simulink model "Joystick"  (Simulink 7.7)
settings: Solver=ode45  StartTime=0.0  StopTime=inf  FixedStep=sample_time  RelTol=1e-3
InitFcn:
  | sample_time=0.01;
libraries: vrlib x7, simulink_extras x5, HDI_Library x2, nid_lib x2, utility x1
settings Model: Creator=ttcl3  LastModifiedBy=CHIEW
settings SolverCC: MaxConsecutiveMinStep=auto
settings DebuggingCC: MultiTaskRateTransMsg=warning

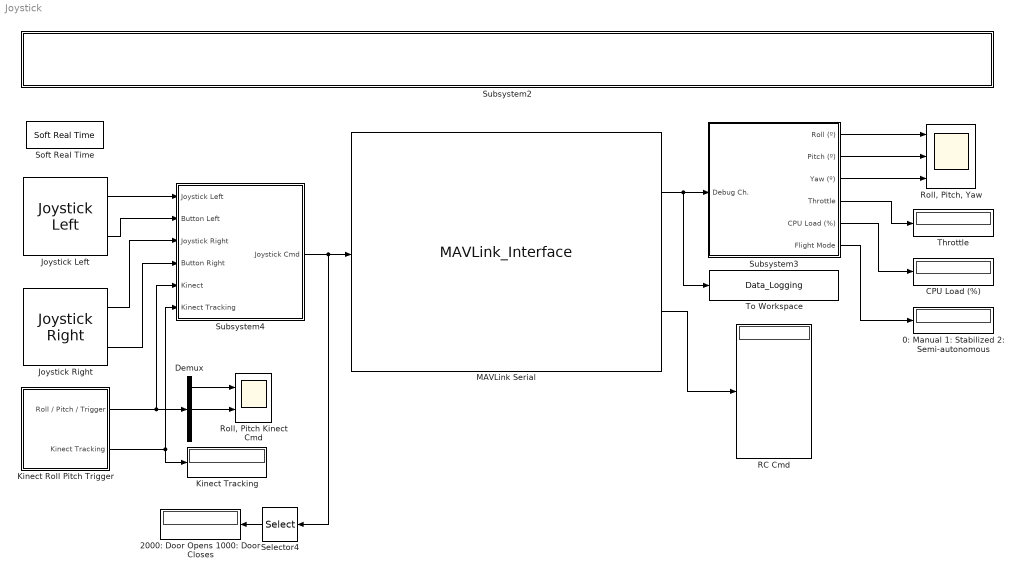
== system Joystick ==
  0: Manual 1: Stabilized 2: Semi-autonomous : Display
  2000: Door Opens 1000: Door Closes : Display
  CPU Load (%) : Display
  Demux : Demux  Outputs=3
  Joystick Left : HDI_Library/Joystick Left  joyid=2  adjustports=on  forcefeed=off
  Joystick Right : HDI_Library/Joystick Right  joyid=1  adjustports=on  forcefeed=off
  Kinect Roll Pitch Trigger : Subsystem
      mask Display: image(imread('kinect.jpg'));port_label('output', 1, 'Roll/Pitch/Trigger'); port_label('output', 2, 'Tracking');
  Kinect Tracking : Display
  MAVLink Serial : S-Function  FunctionName=MAVLink_Interface  Parameters=COM_Port,Baud_Rate,MSG_INPUT,MSG_OUTPUT  EnableBusSupport=off  mask{COM_Port='COM8', Baud_Rate=57600, HEART_BEAT=off, ATTITUDE_OUT=on, RAW_IMU=off, POSITION_OUT=off, VFR_HUD=off, RC_SCALED=on, SERVO_OUT_RAW=off, VICON_XYZ_RPY_Output=off, SET_MODE=off, DATA_STREAM=off, ATTITUDE_COMMAND=off, ATTITUDE_IN=off, GPS_RAW_IN=off, VFR_HUD_IN=off, VICON_XYZ_RPY=on, VICON_VEL=off, POSITION_DESIRED=off}
      mask prompts: COM_Port "COM Port"; Baud_Rate "Baud Rate"; HEART_BEAT "HEART BEAT"; ATTITUDE_OUT "ATTITUDE"; RAW_IMU "RAW IMU"; POSITION_OUT "GLOBAL POSITION"; VFR_HUD "VFR HUD"; RC_SCALED "RC CHANNELS SCALED"; SERVO_OUT_RAW "SERVO OUTPUT RAW"; VICON_XYZ_RPY_Output "VICON Output"; SET_MODE "SET MODE"; DATA_STREAM "REQUEST DATA STREAM"; ATTITUDE_COMMAND "ATTITUDE COMMAND"; ATTITUDE_IN "ATTITUDE (HIL)"; GPS_RAW_IN "GPS RAW (HIL)"; VFR_HUD_IN "AIRSPEED (HIL)"; VICON_XYZ_RPY "VICON POSITION"; VICON_VEL "VICON SPEED"; POSITION_DESIRED "Position Desired"
      mask init:
      | MSG_ID_NUM_INPUT = [uint8(11) uint8(66) uint8(59) uint8(30) uint8(32) uint8(73) uint8(104) uint8(103) uint8(50)];
      | MSG_ID_NAME_INPUT = [SET_MODE DATA_STREAM ATTITUDE_COMMAND ATTITUDE_IN GPS_RAW_IN VFR_HUD_IN VICON_XYZ_RPY VICON_VEL POSITION_DESIRED];
      | 
      | MSG_ID_NUM_OUTPUT = [uint8(0) uint8(30) uint8(27) uint8(73) uint8(74) uint8(34) uint8(37) uint8(104)];
      | MSG_ID_NAME_OUTPUT = [HEART_BEAT ATTITUDE_OUT RAW_IMU VFR_HUD POSITION_OUT RC_SCALED SERVO_OUT_RAW VICON_XYZ_RPY_Output];
      | 
      | idx_input = find(MSG_ID_NAME_INPUT);
      | MSG_INPUT = MSG_ID_NUM_INPUT(idx_input);
      | 
      | idx_output = find(MSG_ID_NAME_OUTPUT);
      | MSG_OUTPUT = MSG_ID_NUM_OUTPUT(idx_output);
      mask TabNameString: Setting,Setting,Output Message,Output Message,Output Message,Output Message,Output Message,Output Message,Output Message,Output Message,Input Message,Input Message,Input Message,Input Message,Input Message,Input Message,Input Message,Input Message,Input Message
      mask Display:
      | % Block image
      | image(imread('10-inch Quad Heat Map.png'));
      | 
      | %Label block
      | fprintf('MAVLink Serial\n%s\n%dbps', COM_Port,  Baud_Rate)
      | 
      | 
      | %Label input ports
      | 
      | in = 1;
      | if (SET_MODE == 1)
      |     port_label('input', in, 'SET MODE');
      |     in = in + 1;
      | end
      | if (DATA_STREAM == 1)
      |     port_label('input', in, 'REQUEST DATA STREAM');
      |     in = in + 1;
      | end
      | if (ATTITUDE_COMMAND == 1)
      |     port_label('input', in, 'ATTITUDE COMMAND');
      |     in = in + 1;
      | end
      | if (ATTITUDE_IN == 1)
      |     port_label('input', in, 'ATTITUDE (HIL)');
      |     in = in + 1;
      | end
      | if (GPS_RAW_IN == 1)
      |     port_label('input', in, 'GPS RAW (HIL)');
      |     in = in + 1;
      | end
      | if (VFR_HUD_IN == 1)
      |     port_label('input', in, 'AIRSPEED (HIL)');
      |     in = in + 1;
      | end
      | if (VICON_XYZ_RPY == 1)
      |     port_label('input', in, 'JOYSTICK CMD');
      |     in = in + 1;
      | end
      | if (VICON_VEL == 1)
      |     port_label('input', in, 'VICON_VEL');
      |     in = in + 1;
      | end
      | 
      | if (POSITION_DESIRED == 1)
      |     port_label('input', in, 'POSITION_DESIRED');
      |     in = in + 1;
      | end
      | 
      | %Label output ports
      | 
      | out = 1;
      | if (HEART_BEAT == 1)
      |     port_label('output', out, 'HEART BEAT');
      |     out = out + 1;
      | end
      | if (ATTITUDE_OUT == 1)
      |     port_label('output', out, 'DEBUG');
      |     out = out + 1;
      | end
      | if (RAW_IMU == 1)
      |     port_label('output', out, 'RAW IMU');
      |     out = out + 1;
      | end
      | if (POSITION_OUT == 1)
      |     port_label('output', out, 'GLOBAL POSITION');
      |     out = out + 1;
      | end
      | if (VFR_HUD == 1)
      |     port_label('output', out, 'VFR HUD');
      |     out = out + 1;
      | end
      | if (RC_SCALED == 1)
      |     port_label('output', out, 'RC CMD');
      |     out = out + 1;
      | end
      | if (SERVO_OUT_RAW == 1)
      |     port_label('output', out, 'SERVO OUTPUT RAW');
      |     out = out + 1;
      | end
      | % weihua, vicon output
      | if (VICON_XYZ_RPY_Output == 1)
      |     port_label('output', out, 'VICON_XYZ_RPY');
      |     out = out + 1;
      | end
  RC Cmd : Display
  "Roll, Pitch Kinect Cmd" : Scope  NumInputPorts=2
      settings: TickLabels=on  TimeRange=24  YMin=-90~-90  YMax=90~90  SampleInput=on
  "Roll, Pitch, Yaw" : Scope  NumInputPorts=3
      settings: TickLabels=on  TimeRange=24  YMin=-90~-90~-90  YMax=90~90~90  SampleInput=on
  Selector4 : Selector  InputPortWidth=7  IndexOptions=Index vector (dialog)  Indices=3  OutputSizes=1
  Soft Real Time : utility/Soft Real Time  x=0.8
  Subsystem2 : Subsystem
      mask Display:
      | %Label block
      | fprintf('NANYANG TECHNOLOGICAL UNIVERSITY')
  Subsystem3 : Subsystem
  Subsystem4 : Subsystem
  Throttle : Display
  To Workspace : ToWorkspace  VariableName=Data_Logging  SampleTime=-1  SaveFormat=Structure With Time
  wires:
  MAVLink Serial/2 -> RC Cmd/1
  Subsystem3/1(Roll (º)) -> "Roll, Pitch, Yaw"/1
  Subsystem3/2(Pitch (º)) -> "Roll, Pitch, Yaw"/2
  Subsystem3/3(Yaw (º)) -> "Roll, Pitch, Yaw"/3
  Subsystem3/4(Throttle) -> Throttle/1
  Subsystem3/5(CPU Load (%)) -> CPU Load (%)/1
  Subsystem3/6(Flight Mode) -> 0: Manual 1: Stabilized 2: Semi-autonomous/1
  MAVLink Serial/1 -> Subsystem3/1(Debug Ch.), To Workspace/1
  Subsystem4/1(Joystick Cmd) -> MAVLink Serial/1, Selector4/1
  Kinect Roll Pitch Trigger/1(Roll / Pitch / Trigger) -> Subsystem4/5(Kinect), Demux/1
  Selector4/1 -> 2000: Door Opens 1000: Door Closes/1
  Kinect Roll Pitch Trigger/2(Kinect Tracking) -> Kinect Tracking/1, Subsystem4/6(Kinect Tracking)
  Demux/1 -> "Roll, Pitch Kinect Cmd"/1
  Demux/2 -> "Roll, Pitch Kinect Cmd"/2
  Joystick Right/1 -> Subsystem4/3(Joystick Right)
  Joystick Right/2 -> Subsystem4/4(Button Right)
  Joystick Left/1 -> Subsystem4/1(Joystick Left)
  Joystick Left/2 -> Subsystem4/2(Button Left)

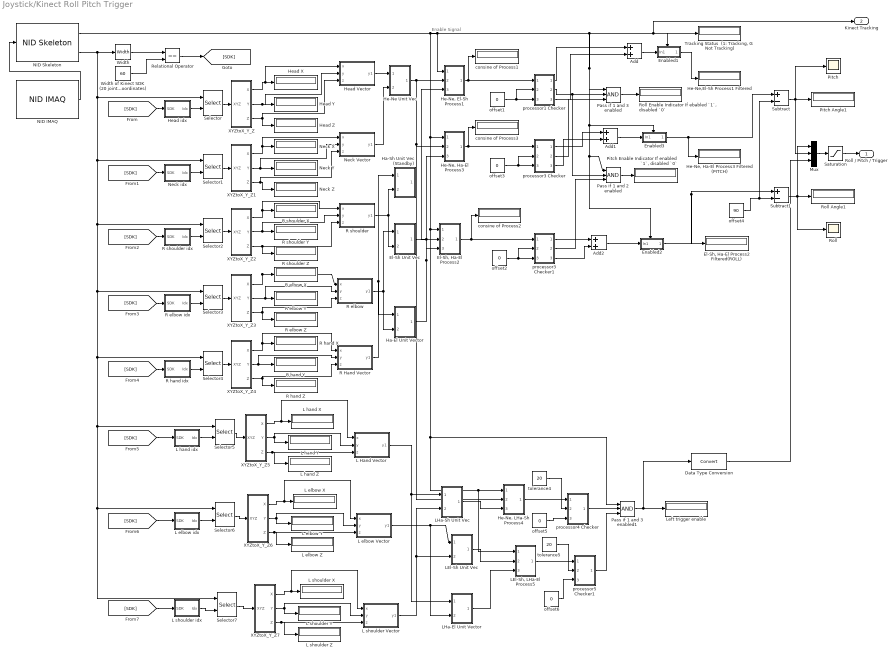
== system Joystick/Kinect Roll Pitch Trigger ==
  note: Enable Signal
  Add : Sum
  Add1 : Sum
  Add2 : Sum
  Data Type Conversion : DataTypeConversion
  El-Sh Unit Vec : Subsystem
  "El-Sh, Ha-El Process2" : Subsystem
  "El-Sh, Ha-El Process2 Filtered(ROLL)" : Display
  Enabled1 : Subsystem  TreatAsAtomicUnit=on
  Enabled2 : Subsystem  TreatAsAtomicUnit=on
  Enabled3 : Subsystem  TreatAsAtomicUnit=on
  Ha-El Unit Vector : Subsystem
  Ha-Sh Unit Vec (Standby) : Subsystem
  He-Ne Unit Vec : Subsystem
  "He-Ne, El-Sh Process1" : Subsystem
  "He-Ne, Ha-El Process3" : Subsystem
  "He-Ne, Ha-El Process3 Filtered (PITCH)" : Display
  "He-Ne, LHa-Sh Process4" : Subsystem
  "He-Ne,El-Sh Process1 Filtered " : Display
  Head Vector : Stateflow chart  TreatAsAtomicUnit=on
  Head X : Display
  Head Y : Display
  Head Z : Display
  Head idx : Subsystem
  L Hand Vector : Stateflow chart  TreatAsAtomicUnit=on
  L elbow Vector : Stateflow chart  TreatAsAtomicUnit=on
  L elbow X : Display
  L elbow Y : Display
  L elbow Z : Display
  L elbow idx : Subsystem
  L hand X : Display
  L hand Y : Display
  L hand Z : Display
  L hand idx : Subsystem
  L shoulder Vector : Stateflow chart  TreatAsAtomicUnit=on
  L shoulder X : Display
  L shoulder Y : Display
  L shoulder Z : Display
  L shoulder idx : Subsystem
  LEl-Sh Unit Vec : Subsystem
  "LEl-Sh, LHa-El Process5" : Subsystem
  LHa-El Unit Vector : Subsystem
  LHa-Sh Unit Vec : Subsystem
  Left trigger enable : Display
  Mux : Mux  Inputs=3
  NID IMAQ : nid_lib/NID IMAQ  imaq_depth=off  imaq_motion=off  imaq_image=off  view_point=off  imaq_skeleton=on  imaq_ir=off  mirror_image=off  imaq_sample_time=1/30  res_fps=VGA (640x480): 30 FPS  needPsiPose=off  angle_input=off  angle=0  angle_read=off  near_mode=off  seated_mode=off  skeleton_smooth=[0.5 0.5 0.5 0.05 0.04]  infer_skeleton=on
  NID Skeleton : nid_lib/NID Skeleton  num_of_skeleton_tracking=1  conv_XYZ_RW=on  viewer=off
  Neck Vector : Stateflow chart  TreatAsAtomicUnit=on
  Neck X : Display
  Neck Y : Display
  Neck Z : Display
  Neck idx : Subsystem
  Pass if 1 and 2 enabled : Logic  Inputs=3  AllPortsSameDT=off  OutDataTypeStr=boolean
  Pass if 1 and 3 enabled : Logic  Inputs=3  AllPortsSameDT=off  OutDataTypeStr=boolean
  Pass if 1 and 3 enabled1 : Logic  Inputs=3  AllPortsSameDT=off  OutDataTypeStr=boolean
  Pitch : Scope
      settings: YMin=-90  YMax=90  SaveName=ScopeData3
  Pitch Angle1 : Display
  "Pitch Enable Indicator If enabled `1`, disabled `0` " : Display
  R Hand Vector : Stateflow chart  TreatAsAtomicUnit=on
  R elbow : Stateflow chart  TreatAsAtomicUnit=on
  R elbow X : Display
  R elbow Y : Display
  R elbow Z : Display
  R elbow idx : Subsystem
  R hand X : Display
  R hand Y : Display
  R hand Z : Display
  R hand idx : Subsystem
  R shoulder : Stateflow chart  TreatAsAtomicUnit=on
  R shoulder X : Display
  R shoulder Y : Display
  R shoulder Z : Display
  R shoulder idx : Subsystem
  Relational Operator : RelationalOperator  Operator===  OutDataTypeStr=boolean
  Roll : Scope
      settings: YMin=-90  YMax=90  SaveName=ScopeData2
  Roll Angle1 : Display
  "Roll Enable Indicator If ebabled `1`, disabled `0`" : Display
  Saturation : Saturate  UpperLimit=30  LowerLimit=-30
  Selector{,1..7} (8 alike) : Selector  NumberOfDimensions=3  InputPortWidth=3  IndexOptions=Select all,Index vector (port),Select all  Indices=[1 3],1,1  OutputSizes=1,1,1
  Subtract : Sum  Inputs=+-
  Subtract1 : Sum  Inputs=+-
  "Tracking Status  (1: Tracking, 0: Not Tracking)" : Display
  Width : Width
  Width of Kinect SDK  (20 joints x 3 coordinates) : Constant  Value=60
  XYZtoX_Y_Z : Subsystem
  XYZtoX_Y_Z1 : Subsystem
  XYZtoX_Y_Z2 : Subsystem
  XYZtoX_Y_Z3 : Subsystem
  XYZtoX_Y_Z4 : Subsystem
  XYZtoX_Y_Z5 : Subsystem
  XYZtoX_Y_Z6 : Subsystem
  XYZtoX_Y_Z7 : Subsystem
  consine of Process1 : Display
  consine of Process2 : Display
  consine of Process3 : Display
  offset{1..3,5..6} (5 alike) : Constant  Value=0
  offset4 : Constant  Value=90
  processor1 Checker : Subsystem
  processor3 Checker : Subsystem
  processor3 Checker1 : Subsystem
  processor4 Checker : Subsystem
  processor5 Checker1 : Subsystem
  tolerance4 : Constant  Value=20
  tolerance5 : Constant  Value=20
  Roll / Pitch / Trigger : Outport
  Kinect Tracking : Outport  Port=2
  wires:
  Saturation/1 -> Roll / Pitch / Trigger/1
  Mux/1 -> Saturation/1
  Pass if 1 and 3 enabled/1 -> "Roll Enable Indicator If ebabled `1`, disabled `0`"/1
  Subtract1/1 -> Roll/1, Mux/1, Roll Angle1/1
  Subtract/1 -> Pitch/1, Mux/2, Pitch Angle1/1
  offset4/1 -> Subtract/2, Subtract1/2
  Add2/1 -> Enabled2/1(In1)
  processor3 Checker1/3(Out3) -> Add2/2
  processor3 Checker1/1(Out1) -> Add2/1
  processor3 Checker/3(Out3) -> Add1/2
  processor3 Checker/1(Out1) -> Add1/1
  Add1/1 -> Enabled3/1(In1)
  processor1 Checker/1(Out1) -> Add/1
  Add/1 -> Enabled1/1(In1)
  processor1 Checker/3(Out3) -> Add/2
  Enabled2/1(Out1) -> Subtract1/1, "El-Sh, Ha-El Process2 Filtered(ROLL)"/1
  Enabled1/1(Out1) -> "He-Ne,El-Sh Process1 Filtered "/1
  Enabled3/1(Out1) -> Subtract/1, "He-Ne, Ha-El Process3 Filtered (PITCH)"/1
  offset2/1 -> processor3 Checker1/2(In2), processor3 Checker1/3(In3)
  offset3/1 -> processor3 Checker/2(In2), processor3 Checker/3(In3)
  offset1/1 -> processor1 Checker/2(In2), processor1 Checker/3(In3)
  processor3 Checker1/2(Out2) -> Pass if 1 and 2 enabled/3
  processor1 Checker/2(Out2) -> Pass if 1 and 2 enabled/2, Pass if 1 and 3 enabled/2
  processor3 Checker/2(Out2) -> Pass if 1 and 3 enabled/3
  Pass if 1 and 2 enabled/1 -> "Pitch Enable Indicator If enabled `1`, disabled `0` "/1
  "El-Sh, Ha-El Process2"/1(Out1) -> processor3 Checker1/1(In1), consine of Process2/1
  "He-Ne, El-Sh Process1"/1(Out1) -> consine of Process1/1, processor1 Checker/1(In1)
  "He-Ne, Ha-El Process3"/1(Out1) -> processor3 Checker/1(In1), consine of Process3/1
  Ha-El Unit Vector/1(Out1) -> "He-Ne, Ha-El Process3"/3(In3), "El-Sh, Ha-El Process2"/3(In3)
  El-Sh Unit Vec/1(Out1) -> "El-Sh, Ha-El Process2"/2(In2), "He-Ne, El-Sh Process1"/3(In3)
  He-Ne Unit Vec/1(Out1) -> "He-Ne, El-Sh Process1"/2(In2), "He-Ne, Ha-El Process3"/2(In2), "He-Ne, LHa-Sh Process4"/2(In2)
  R elbow/1(y1) -> Ha-El Unit Vector/2(In2), El-Sh Unit Vec/1(In1)
  R Hand Vector/1(y1) -> Ha-El Unit Vector/1(In1), Ha-Sh Unit Vec (Standby)/1(In1)
  R shoulder/1(y1) -> El-Sh Unit Vec/2(In2), Ha-Sh Unit Vec (Standby)/2(In2)
  Head Vector/1(y1) -> He-Ne Unit Vec/1(In1)
  Neck Vector/1(y1) -> He-Ne Unit Vec/2(In2)
  Selector/1 -> XYZtoX_Y_Z/1(XYZ)
  Selector4/1 -> XYZtoX_Y_Z4/1(XYZ)
  XYZtoX_Y_Z4/3(Z) -> R Hand Vector/3(z), R hand Z/1
  XYZtoX_Y_Z4/2(Y) -> R Hand Vector/2(y), R hand Y/1
  XYZtoX_Y_Z4/1(X) -> R Hand Vector/1(x), R hand X/1
  Selector3/1 -> XYZtoX_Y_Z3/1(XYZ)
  XYZtoX_Y_Z3/3(Z) -> R elbow/3(z), R elbow Z/1
  XYZtoX_Y_Z3/2(Y) -> R elbow/2(y), R elbow Y/1
  XYZtoX_Y_Z3/1(X) -> R elbow/1(x), R elbow X/1
  Selector2/1 -> XYZtoX_Y_Z2/1(XYZ)
  XYZtoX_Y_Z2/3(Z) -> R shoulder/3(z), R shoulder Z/1
  XYZtoX_Y_Z2/2(Y) -> R shoulder/2(y), R shoulder Y/1
  XYZtoX_Y_Z2/1(X) -> R shoulder/1(x), R shoulder X/1
  XYZtoX_Y_Z1/3(Z) -> Neck Vector/3(z), Neck Z/1
  XYZtoX_Y_Z1/2(Y) -> Neck Vector/2(y), Neck Y/1
  XYZtoX_Y_Z1/1(X) -> Neck Vector/1(x), Neck X/1
  XYZtoX_Y_Z/3(Z) -> Head Vector/3(z), Head Z/1
  XYZtoX_Y_Z/2(Y) -> Head Vector/2(y), Head Y/1
  [SDK] -> R hand idx/1(SDK)
  R hand idx/1(Idx) -> Selector4/2
  [SDK] -> R elbow idx/1(SDK)
  R elbow idx/1(Idx) -> Selector3/2
  [SDK] -> R shoulder idx/1(SDK)
  R shoulder idx/1(Idx) -> Selector2/2
  Selector1/1 -> XYZtoX_Y_Z1/1(XYZ)
  [SDK] -> Neck idx/1(SDK)
  Neck idx/1(Idx) -> Selector1/2
  XYZtoX_Y_Z/1(X) -> Head Vector/1(x), Head X/1
  NID Skeleton/1 -> "He-Ne, El-Sh Process1"/1(In1), Pass if 1 and 3 enabled/1, Kinect Tracking/1, "Tracking Status  (1: Tracking, 0: Not Tracking)"/1, Enabled1/Enable, Enabled3/Enable, Enabled2/Enable, Pass if 1 and 2 enabled/1, "He-Ne, Ha-El Process3"/1(In1), "El-Sh, Ha-El Process2"/1(In1), "He-Ne, LHa-Sh Process4"/1(In1), "LEl-Sh, LHa-El Process5"/1(In1), Pass if 1 and 3 enabled1/1
  [SDK] -> Head idx/1(SDK)
  Head idx/1(Idx) -> Selector/2
  Relational Operator/1 -> [SDK]
  NID Skeleton/2 -> Selector3/1, Selector4/1, Selector5/1, Selector6/1, Selector7/1, Selector2/1, Selector1/1, Selector/1, Width/1
  Width of Kinect SDK  (20 joints x 3 coordinates)/1 -> Relational Operator/2
  Width/1 -> Relational Operator/1
  NID IMAQ/1 -> NID Skeleton/1
  [SDK] -> L hand idx/1(SDK)
  [SDK] -> L elbow idx/1(SDK)
  [SDK] -> L shoulder idx/1(SDK)
  L hand idx/1(Idx) -> Selector5/2
  L elbow idx/1(Idx) -> Selector6/2
  L shoulder idx/1(Idx) -> Selector7/2
  Selector5/1 -> XYZtoX_Y_Z5/1(XYZ)
  XYZtoX_Y_Z5/1(X) -> L hand X/1, L Hand Vector/1(x)
  XYZtoX_Y_Z5/2(Y) -> L hand Y/1, L Hand Vector/2(y)
  XYZtoX_Y_Z5/3(Z) -> L hand Z/1, L Hand Vector/3(z)
  XYZtoX_Y_Z6/1(X) -> L elbow X/1, L elbow Vector/1(x)
  XYZtoX_Y_Z6/2(Y) -> L elbow Y/1, L elbow Vector/2(y)
  XYZtoX_Y_Z6/3(Z) -> L elbow Z/1, L elbow Vector/3(z)
  XYZtoX_Y_Z7/1(X) -> L shoulder X/1, L shoulder Vector/1(x)
  XYZtoX_Y_Z7/2(Y) -> L shoulder Y/1, L shoulder Vector/2(y)
  XYZtoX_Y_Z7/3(Z) -> L shoulder Z/1, L shoulder Vector/3(z)
  Selector6/1 -> XYZtoX_Y_Z6/1(XYZ)
  L Hand Vector/1(y1) -> LHa-Sh Unit Vec/1(In1), LHa-El Unit Vector/1(In1)
  L shoulder Vector/1(y1) -> LHa-Sh Unit Vec/2(In2), LEl-Sh Unit Vec/2(In2)
  LHa-Sh Unit Vec/1(Out1) -> "He-Ne, LHa-Sh Process4"/3(In3)
  "He-Ne, LHa-Sh Process4"/1(Out1) -> processor4 Checker/1(In1)
  tolerance4/1 -> processor4 Checker/2(In2)
  offset5/1 -> processor4 Checker/3(In3)
  Selector7/1 -> XYZtoX_Y_Z7/1(XYZ)
  processor4 Checker/1(Out2) -> Pass if 1 and 3 enabled1/2
  L elbow Vector/1(y1) -> LEl-Sh Unit Vec/1(In1), LHa-El Unit Vector/2(In2)
  LEl-Sh Unit Vec/1(Out1) -> "LEl-Sh, LHa-El Process5"/2(In2)
  LHa-El Unit Vector/1(Out1) -> "LEl-Sh, LHa-El Process5"/3(In3)
  "LEl-Sh, LHa-El Process5"/1(Out1) -> processor5 Checker1/1(In1)
  tolerance5/1 -> processor5 Checker1/2(In2)
  offset6/1 -> processor5 Checker1/3(In3)
  processor5 Checker1/1(Out2) -> Pass if 1 and 3 enabled1/3
  Pass if 1 and 3 enabled1/1 -> Left trigger enable/1, Data Type Conversion/1
  Data Type Conversion/1 -> Mux/3

== system Joystick/Subsystem2 ==

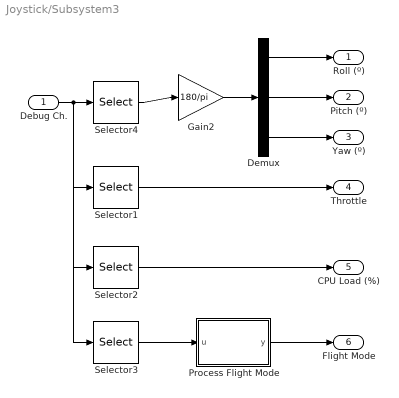
== system Joystick/Subsystem3 ==
  Debug Ch. : Inport
  Demux : Demux  Outputs=3
  Gain2 : Gain  Gain=180/pi
  Process Flight Mode : Stateflow chart  TreatAsAtomicUnit=on
  Selector1 : Selector  InputPortWidth=6  IndexOptions=Index vector (dialog)  Indices=4  OutputSizes=1
  Selector2 : Selector  InputPortWidth=6  IndexOptions=Index vector (dialog)  Indices=5  OutputSizes=1
  Selector3 : Selector  InputPortWidth=6  IndexOptions=Index vector (dialog)  Indices=6  OutputSizes=1
  Selector4 : Selector  InputPortWidth=6  IndexOptions=Index vector (dialog)  Indices=[1 2 3]  OutputSizes=1
  Roll (º) : Outport
  Pitch (º) : Outport  Port=2
  Yaw (º) : Outport  Port=3
  Throttle : Outport  Port=4
  CPU Load (%) : Outport  Port=5
  Flight Mode : Outport  Port=6
  wires:
  Selector4/1 -> Gain2/1
  Gain2/1 -> Demux/1
  Demux/1 -> Roll (º)/1
  Demux/2 -> Pitch (º)/1
  Debug Ch./1 -> Selector4/1, Selector1/1, Selector2/1, Selector3/1
  Demux/3 -> Yaw (º)/1
  Selector1/1 -> Throttle/1
  Selector2/1 -> CPU Load (%)/1
  Selector3/1 -> Process Flight Mode/1(u)
  Process Flight Mode/1(y) -> Flight Mode/1

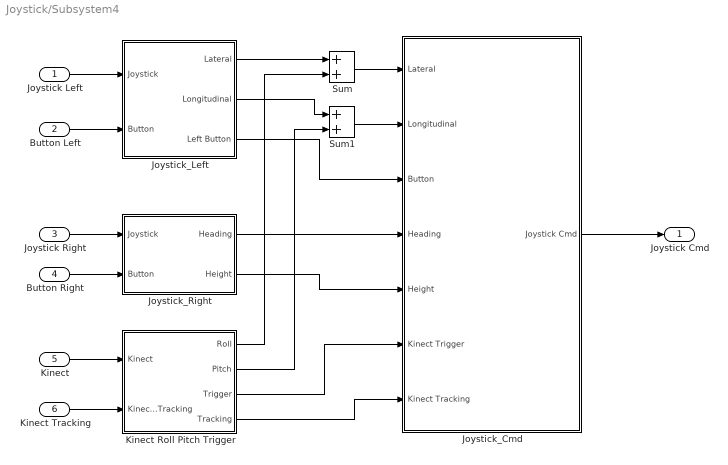
== system Joystick/Subsystem4 ==
  Joystick Left : Inport
  Button Left : Inport  Port=2
  Joystick Right : Inport  Port=3
  Button Right : Inport  Port=4
  Kinect : Inport  Port=5
  Kinect Tracking : Inport  Port=6
  Joystick_Cmd : Subsystem
  Joystick_Left : Subsystem
  Joystick_Right : Subsystem
  Kinect Roll Pitch Trigger : Subsystem
  Sum : Sum
  Sum1 : Sum
  Joystick Cmd : Outport
  wires:
  Joystick Left/1 -> Joystick_Left/1(Joystick)
  Joystick Right/1 -> Joystick_Right/1(Joystick)
  Button Right/1 -> Joystick_Right/2(Button)
  Button Left/1 -> Joystick_Left/2(Button)
  Joystick_Right/1(Heading) -> Joystick_Cmd/4(Heading)
  Joystick_Right/2(Height) -> Joystick_Cmd/5(Height)
  Kinect/1 -> Kinect Roll Pitch Trigger/1(Kinect)
  Joystick_Left/3(Left Button) -> Joystick_Cmd/3(Button)
  Joystick_Cmd/1(Joystick Cmd) -> Joystick Cmd/1
  Joystick_Left/1(Lateral) -> Sum/1
  Sum/1 -> Joystick_Cmd/1(Lateral)
  Sum1/1 -> Joystick_Cmd/2(Longitudinal)
  Joystick_Left/2(Longitudinal) -> Sum1/1
  Kinect Roll Pitch Trigger/3(Trigger) -> Joystick_Cmd/6(Kinect Trigger)
  Kinect Tracking/1 -> Kinect Roll Pitch Trigger/2(Kinect Tracking)
  Kinect Roll Pitch Trigger/4(Tracking) -> Joystick_Cmd/7(Kinect Tracking)
  Kinect Roll Pitch Trigger/1(Roll) -> Sum/2
  Kinect Roll Pitch Trigger/2(Pitch) -> Sum1/2

== system Joystick/Kinect Roll Pitch Trigger/El-Sh Unit Vec ==
  In1 : Inport
  In2 : Inport  Port=2
  Shoudler Elbow : vrlib/Utilities/Normalize Vector  SystemSampleTime=-1  maxzero=0
  Subtract3 : Sum  Inputs=+-
  Out1 : Outport
  wires:
  Shoudler Elbow/1 -> Out1/1
  In2/1 -> Subtract3/2
  In1/1 -> Subtract3/1
  Subtract3/1 -> Shoudler Elbow/1

== system Joystick/Kinect Roll Pitch Trigger/El-Sh, Ha-El Process2 ==
  In1 : Inport
  In2 : Inport  Port=2
  In3 : Inport  Port=3
  Enabled Subsystem2 : Subsystem  TreatAsAtomicUnit=on
  "consine El-Sh, Ha-El" : DotProduct  InputSameDT=on  OutDataTypeStr=Inherit: Inherit via internal rule
  Out1 : Outport
  wires:
  Enabled Subsystem2/1(Out1) -> Out1/1
  In3/1 -> "consine El-Sh, Ha-El"/2
  In2/1 -> "consine El-Sh, Ha-El"/1
  In1/1 -> Enabled Subsystem2/Enable
  "consine El-Sh, Ha-El"/1 -> Enabled Subsystem2/1(In1)

== system Joystick/Kinect Roll Pitch Trigger/Enabled1 ==
  In1 : Inport
  Enable : EnablePort
  Out1 : Outport
  wires:
  In1/1 -> Out1/1

== system Joystick/Kinect Roll Pitch Trigger/Enabled2 ==
  In1 : Inport
  Enable : EnablePort
  Out1 : Outport
  wires:
  In1/1 -> Out1/1

== system Joystick/Kinect Roll Pitch Trigger/Enabled3 ==
  In1 : Inport
  Enable : EnablePort
  Out1 : Outport
  wires:
  In1/1 -> Out1/1

== system Joystick/Kinect Roll Pitch Trigger/Ha-El Unit Vector ==
  In1 : Inport
  In2 : Inport  Port=2
  Elbow Hand : vrlib/Utilities/Normalize Vector  SystemSampleTime=-1  maxzero=0
  Subtract2 : Sum  Inputs=+-
  Out1 : Outport
  wires:
  Elbow Hand/1 -> Out1/1
  In2/1 -> Subtract2/2
  In1/1 -> Subtract2/1
  Subtract2/1 -> Elbow Hand/1

== system Joystick/Kinect Roll Pitch Trigger/Ha-Sh Unit Vec (Standby) ==
  In1 : Inport
  In2 : Inport  Port=2
  Subtract1 : Sum  Inputs=+-
  Unit Vector1 : vrlib/Utilities/Normalize Vector  SystemSampleTime=-1  maxzero=0
  Out1 : Outport
  wires:
  Unit Vector1/1 -> Out1/1
  In2/1 -> Subtract1/2
  In1/1 -> Subtract1/1
  Subtract1/1 -> Unit Vector1/1

== system Joystick/Kinect Roll Pitch Trigger/He-Ne Unit Vec ==
  In1 : Inport
  In2 : Inport  Port=2
  Subtract : Sum  Inputs=+-
  Unit Vector : vrlib/Utilities/Normalize Vector  SystemSampleTime=-1  maxzero=0
  Out1 : Outport
  wires:
  In2/1 -> Subtract/2
  Unit Vector/1 -> Out1/1
  In1/1 -> Subtract/1
  Subtract/1 -> Unit Vector/1

== system Joystick/Kinect Roll Pitch Trigger/He-Ne, El-Sh Process1 ==
  In1 : Inport
  In2 : Inport  Port=2
  In3 : Inport  Port=3
  Enabled Subsystem1 : Subsystem  TreatAsAtomicUnit=on
  consine He-Ne El-Sh : DotProduct  InputSameDT=on  OutDataTypeStr=Inherit: Inherit via internal rule
  Out1 : Outport
  wires:
  Enabled Subsystem1/1(Out1) -> Out1/1
  In3/1 -> consine He-Ne El-Sh/2
  In2/1 -> consine He-Ne El-Sh/1
  In1/1 -> Enabled Subsystem1/Enable
  consine He-Ne El-Sh/1 -> Enabled Subsystem1/1(In1)

== system Joystick/Kinect Roll Pitch Trigger/He-Ne, Ha-El Process3 ==
  In1 : Inport
  In2 : Inport  Port=2
  In3 : Inport  Port=3
  Enabled Subsystem3 : Subsystem  TreatAsAtomicUnit=on
  "consine He-Ne, Ha-El" : DotProduct  InputSameDT=on  OutDataTypeStr=Inherit: Inherit via internal rule
  Out1 : Outport
  wires:
  Enabled Subsystem3/1(Out1) -> Out1/1
  In3/1 -> "consine He-Ne, Ha-El"/2
  In2/1 -> "consine He-Ne, Ha-El"/1
  In1/1 -> Enabled Subsystem3/Enable
  "consine He-Ne, Ha-El"/1 -> Enabled Subsystem3/1(In1)

== system Joystick/Kinect Roll Pitch Trigger/He-Ne, LHa-Sh Process4 ==
  In1 : Inport
  In2 : Inport  Port=2
  In3 : Inport  Port=3
  Enabled Subsystem1 : Subsystem  TreatAsAtomicUnit=on
  consine He-Ne El-Sh : DotProduct  InputSameDT=on  OutDataTypeStr=Inherit: Inherit via internal rule
  Out1 : Outport
  wires:
  consine He-Ne El-Sh/1 -> Enabled Subsystem1/1(In1)
  In1/1 -> Enabled Subsystem1/Enable
  In2/1 -> consine He-Ne El-Sh/1
  In3/1 -> consine He-Ne El-Sh/2
  Enabled Subsystem1/1(Out1) -> Out1/1

== system Joystick/Kinect Roll Pitch Trigger/Head idx ==
  SDK : Inport
  Kinect SDK : Constant  Value=4
  OpenNI : Constant
  Switch : Switch  Criteria=u2 ~= 0
  Idx : Outport
  wires:
  Switch/1 -> Idx/1
  SDK/1 -> Switch/2
  OpenNI/1 -> Switch/3
  Kinect SDK/1 -> Switch/1

== system Joystick/Kinect Roll Pitch Trigger/L elbow idx ==
  SDK : Inport
  Kinect SDK : Constant  Value=6
  OpenNI : Constant  Value=8
  Switch : Switch  Criteria=u2 ~= 0
  Idx : Outport
  wires:
  Kinect SDK/1 -> Switch/1
  OpenNI/1 -> Switch/3
  SDK/1 -> Switch/2
  Switch/1 -> Idx/1

== system Joystick/Kinect Roll Pitch Trigger/L hand idx ==
  SDK : Inport
  Kinect SDK : Constant  Value=8
  OpenNI : Constant  Value=9
  Switch : Switch  Criteria=u2 ~= 0
  Idx : Outport
  wires:
  Kinect SDK/1 -> Switch/1
  OpenNI/1 -> Switch/3
  SDK/1 -> Switch/2
  Switch/1 -> Idx/1

== system Joystick/Kinect Roll Pitch Trigger/L shoulder idx ==
  SDK : Inport
  Kinect SDK : Constant  Value=5
  OpenNI : Constant  Value=7
  Switch : Switch  Criteria=u2 ~= 0
  Idx : Outport
  wires:
  Kinect SDK/1 -> Switch/1
  OpenNI/1 -> Switch/3
  SDK/1 -> Switch/2
  Switch/1 -> Idx/1

== system Joystick/Kinect Roll Pitch Trigger/LEl-Sh Unit Vec ==
  In1 : Inport
  In2 : Inport  Port=2
  Shoudler Elbow : vrlib/Utilities/Normalize Vector  SystemSampleTime=-1  maxzero=0
  Subtract3 : Sum  Inputs=+-
  Out1 : Outport
  wires:
  Subtract3/1 -> Shoudler Elbow/1
  In1/1 -> Subtract3/1
  In2/1 -> Subtract3/2
  Shoudler Elbow/1 -> Out1/1

== system Joystick/Kinect Roll Pitch Trigger/LEl-Sh, LHa-El Process5 ==
  In1 : Inport
  In2 : Inport  Port=2
  In3 : Inport  Port=3
  Enabled Subsystem2 : Subsystem  TreatAsAtomicUnit=on
  "consine El-Sh, Ha-El" : DotProduct  InputSameDT=on  OutDataTypeStr=Inherit: Inherit via internal rule
  Out1 : Outport
  wires:
  "consine El-Sh, Ha-El"/1 -> Enabled Subsystem2/1(In1)
  In1/1 -> Enabled Subsystem2/Enable
  In2/1 -> "consine El-Sh, Ha-El"/1
  In3/1 -> "consine El-Sh, Ha-El"/2
  Enabled Subsystem2/1(Out1) -> Out1/1

== system Joystick/Kinect Roll Pitch Trigger/LHa-El Unit Vector ==
  In1 : Inport
  In2 : Inport  Port=2
  Elbow Hand : vrlib/Utilities/Normalize Vector  SystemSampleTime=-1  maxzero=0
  Subtract2 : Sum  Inputs=+-
  Out1 : Outport
  wires:
  Subtract2/1 -> Elbow Hand/1
  In1/1 -> Subtract2/1
  In2/1 -> Subtract2/2
  Elbow Hand/1 -> Out1/1

== system Joystick/Kinect Roll Pitch Trigger/LHa-Sh Unit Vec ==
  In1 : Inport
  In2 : Inport  Port=2
  Subtract1 : Sum  Inputs=+-
  Unit Vector1 : vrlib/Utilities/Normalize Vector  SystemSampleTime=-1  maxzero=0
  Out1 : Outport
  wires:
  Subtract1/1 -> Unit Vector1/1
  In1/1 -> Subtract1/1
  In2/1 -> Subtract1/2
  Unit Vector1/1 -> Out1/1

== system Joystick/Kinect Roll Pitch Trigger/Neck idx ==
  SDK : Inport
  Kinect SDK : Constant  Value=3
  OpenNI : Constant  Value=2
  Switch : Switch  Criteria=u2 ~= 0
  Idx : Outport
  wires:
  Kinect SDK/1 -> Switch/1
  OpenNI/1 -> Switch/3
  SDK/1 -> Switch/2
  Switch/1 -> Idx/1

== system Joystick/Kinect Roll Pitch Trigger/R elbow idx ==
  SDK : Inport
  Kinect SDK : Constant  Value=10
  OpenNI : Constant  Value=5
  Switch : Switch  Criteria=u2 ~= 0
  Idx : Outport
  wires:
  Switch/1 -> Idx/1
  SDK/1 -> Switch/2
  OpenNI/1 -> Switch/3
  Kinect SDK/1 -> Switch/1

== system Joystick/Kinect Roll Pitch Trigger/R hand idx ==
  SDK : Inport
  Kinect SDK : Constant  Value=12
  OpenNI : Constant  Value=6
  Switch : Switch  Criteria=u2 ~= 0
  Idx : Outport
  wires:
  Switch/1 -> Idx/1
  SDK/1 -> Switch/2
  OpenNI/1 -> Switch/3
  Kinect SDK/1 -> Switch/1

== system Joystick/Kinect Roll Pitch Trigger/R shoulder idx ==
  SDK : Inport
  Kinect SDK : Constant  Value=9
  OpenNI : Constant  Value=4
  Switch : Switch  Criteria=u2 ~= 0
  Idx : Outport
  wires:
  Switch/1 -> Idx/1
  SDK/1 -> Switch/2
  OpenNI/1 -> Switch/3
  Kinect SDK/1 -> Switch/1

== system Joystick/Kinect Roll Pitch Trigger/XYZtoX_Y_Z ==
  XYZ : Inport
  Selector : Selector  NumberOfDimensions=3  InputPortWidth=3  IndexOptions=Index vector (dialog),Index vector (dialog),Index vector (dialog)  Indices=1,1,1  OutputSizes=1,1,1
  Selector1 : Selector  NumberOfDimensions=3  InputPortWidth=3  IndexOptions=Index vector (dialog),Index vector (dialog),Index vector (dialog)  Indices=1,1,2  OutputSizes=1,1,1
  Selector2 : Selector  NumberOfDimensions=3  InputPortWidth=3  IndexOptions=Index vector (dialog),Index vector (dialog),Index vector (dialog)  Indices=1,1,3  OutputSizes=1,1,1
  X : Outport
  Y : Outport  Port=2
  Z : Outport  Port=3
  wires:
  Selector2/1 -> Z/1
  Selector1/1 -> Y/1
  Selector/1 -> X/1
  XYZ/1 -> Selector2/1, Selector1/1, Selector/1

== system Joystick/Kinect Roll Pitch Trigger/XYZtoX_Y_Z1 ==
  XYZ : Inport
  Selector : Selector  NumberOfDimensions=3  InputPortWidth=3  IndexOptions=Index vector (dialog),Index vector (dialog),Index vector (dialog)  Indices=1,1,1  OutputSizes=1,1,1
  Selector1 : Selector  NumberOfDimensions=3  InputPortWidth=3  IndexOptions=Index vector (dialog),Index vector (dialog),Index vector (dialog)  Indices=1,1,2  OutputSizes=1,1,1
  Selector2 : Selector  NumberOfDimensions=3  InputPortWidth=3  IndexOptions=Index vector (dialog),Index vector (dialog),Index vector (dialog)  Indices=1,1,3  OutputSizes=1,1,1
  X : Outport
  Y : Outport  Port=2
  Z : Outport  Port=3
  wires:
  XYZ/1 -> Selector/1, Selector1/1, Selector2/1
  Selector/1 -> X/1
  Selector1/1 -> Y/1
  Selector2/1 -> Z/1

== system Joystick/Kinect Roll Pitch Trigger/XYZtoX_Y_Z2 ==
  XYZ : Inport
  Selector : Selector  NumberOfDimensions=3  InputPortWidth=3  IndexOptions=Index vector (dialog),Index vector (dialog),Index vector (dialog)  Indices=1,1,1  OutputSizes=1,1,1
  Selector1 : Selector  NumberOfDimensions=3  InputPortWidth=3  IndexOptions=Index vector (dialog),Index vector (dialog),Index vector (dialog)  Indices=1,1,2  OutputSizes=1,1,1
  Selector2 : Selector  NumberOfDimensions=3  InputPortWidth=3  IndexOptions=Index vector (dialog),Index vector (dialog),Index vector (dialog)  Indices=1,1,3  OutputSizes=1,1,1
  X : Outport
  Y : Outport  Port=2
  Z : Outport  Port=3
  wires:
  Selector2/1 -> Z/1
  Selector1/1 -> Y/1
  Selector/1 -> X/1
  XYZ/1 -> Selector2/1, Selector1/1, Selector/1

== system Joystick/Kinect Roll Pitch Trigger/XYZtoX_Y_Z3 ==
  XYZ : Inport
  Selector : Selector  NumberOfDimensions=3  InputPortWidth=3  IndexOptions=Index vector (dialog),Index vector (dialog),Index vector (dialog)  Indices=1,1,1  OutputSizes=1,1,1
  Selector1 : Selector  NumberOfDimensions=3  InputPortWidth=3  IndexOptions=Index vector (dialog),Index vector (dialog),Index vector (dialog)  Indices=1,1,2  OutputSizes=1,1,1
  Selector2 : Selector  NumberOfDimensions=3  InputPortWidth=3  IndexOptions=Index vector (dialog),Index vector (dialog),Index vector (dialog)  Indices=1,1,3  OutputSizes=1,1,1
  X : Outport
  Y : Outport  Port=2
  Z : Outport  Port=3
  wires:
  XYZ/1 -> Selector/1, Selector1/1, Selector2/1
  Selector/1 -> X/1
  Selector1/1 -> Y/1
  Selector2/1 -> Z/1

== system Joystick/Kinect Roll Pitch Trigger/XYZtoX_Y_Z4 ==
  XYZ : Inport
  Selector : Selector  NumberOfDimensions=3  InputPortWidth=3  IndexOptions=Index vector (dialog),Index vector (dialog),Index vector (dialog)  Indices=1,1,1  OutputSizes=1,1,1
  Selector1 : Selector  NumberOfDimensions=3  InputPortWidth=3  IndexOptions=Index vector (dialog),Index vector (dialog),Index vector (dialog)  Indices=1,1,2  OutputSizes=1,1,1
  Selector2 : Selector  NumberOfDimensions=3  InputPortWidth=3  IndexOptions=Index vector (dialog),Index vector (dialog),Index vector (dialog)  Indices=1,1,3  OutputSizes=1,1,1
  X : Outport
  Y : Outport  Port=2
  Z : Outport  Port=3
  wires:
  Selector2/1 -> Z/1
  Selector1/1 -> Y/1
  Selector/1 -> X/1
  XYZ/1 -> Selector2/1, Selector1/1, Selector/1

== system Joystick/Kinect Roll Pitch Trigger/XYZtoX_Y_Z5 ==
  XYZ : Inport
  Selector : Selector  NumberOfDimensions=3  InputPortWidth=3  IndexOptions=Index vector (dialog),Index vector (dialog),Index vector (dialog)  Indices=1,1,1  OutputSizes=1,1,1
  Selector1 : Selector  NumberOfDimensions=3  InputPortWidth=3  IndexOptions=Index vector (dialog),Index vector (dialog),Index vector (dialog)  Indices=1,1,2  OutputSizes=1,1,1
  Selector2 : Selector  NumberOfDimensions=3  InputPortWidth=3  IndexOptions=Index vector (dialog),Index vector (dialog),Index vector (dialog)  Indices=1,1,3  OutputSizes=1,1,1
  X : Outport
  Y : Outport  Port=2
  Z : Outport  Port=3
  wires:
  XYZ/1 -> Selector/1, Selector1/1, Selector2/1
  Selector/1 -> X/1
  Selector1/1 -> Y/1
  Selector2/1 -> Z/1

== system Joystick/Kinect Roll Pitch Trigger/XYZtoX_Y_Z6 ==
  XYZ : Inport
  Selector : Selector  NumberOfDimensions=3  InputPortWidth=3  IndexOptions=Index vector (dialog),Index vector (dialog),Index vector (dialog)  Indices=1,1,1  OutputSizes=1,1,1
  Selector1 : Selector  NumberOfDimensions=3  InputPortWidth=3  IndexOptions=Index vector (dialog),Index vector (dialog),Index vector (dialog)  Indices=1,1,2  OutputSizes=1,1,1
  Selector2 : Selector  NumberOfDimensions=3  InputPortWidth=3  IndexOptions=Index vector (dialog),Index vector (dialog),Index vector (dialog)  Indices=1,1,3  OutputSizes=1,1,1
  X : Outport
  Y : Outport  Port=2
  Z : Outport  Port=3
  wires:
  XYZ/1 -> Selector/1, Selector1/1, Selector2/1
  Selector/1 -> X/1
  Selector1/1 -> Y/1
  Selector2/1 -> Z/1

== system Joystick/Kinect Roll Pitch Trigger/XYZtoX_Y_Z7 ==
  XYZ : Inport
  Selector : Selector  NumberOfDimensions=3  InputPortWidth=3  IndexOptions=Index vector (dialog),Index vector (dialog),Index vector (dialog)  Indices=1,1,1  OutputSizes=1,1,1
  Selector1 : Selector  NumberOfDimensions=3  InputPortWidth=3  IndexOptions=Index vector (dialog),Index vector (dialog),Index vector (dialog)  Indices=1,1,2  OutputSizes=1,1,1
  Selector2 : Selector  NumberOfDimensions=3  InputPortWidth=3  IndexOptions=Index vector (dialog),Index vector (dialog),Index vector (dialog)  Indices=1,1,3  OutputSizes=1,1,1
  X : Outport
  Y : Outport  Port=2
  Z : Outport  Port=3
  wires:
  XYZ/1 -> Selector/1, Selector1/1, Selector2/1
  Selector/1 -> X/1
  Selector1/1 -> Y/1
  Selector2/1 -> Z/1

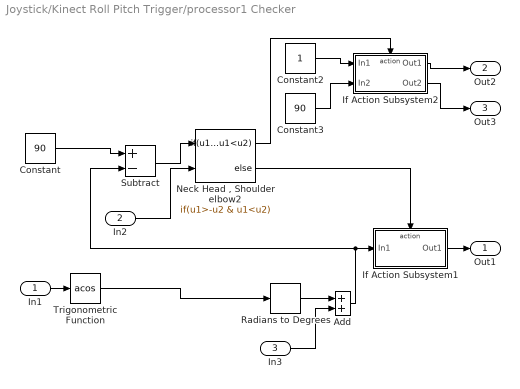
== system Joystick/Kinect Roll Pitch Trigger/processor1 Checker ==
  In1 : Inport
  In2 : Inport  Port=2
  In3 : Inport  Port=3
  Add : Sum
  Constant : Constant  Value=90
  Constant2 : Constant
  Constant3 : Constant  Value=90
  If Action Subsystem1 : Subsystem  TreatAsAtomicUnit=on
  If Action Subsystem2 : Subsystem  TreatAsAtomicUnit=on
  "Neck Head , Shoulder elbow2" : If  NumInputs=2  IfExpression=u1>-u2 & u1<u2
  Radians to Degrees : simulink_extras/Transformations/Radians to Degrees  SystemSampleTime=-1
  Subtract : Sum  Inputs=+-
  Trigonometric Function : Trigonometry  Operator=acos
  Out1 : Outport
  Out2 : Outport  Port=2
  Out3 : Outport  Port=3
  wires:
  If Action Subsystem2/2(Out2) -> Out3/1
  Constant3/1 -> If Action Subsystem2/2(In2)
  Trigonometric Function/1 -> Radians to Degrees/1
  In3/1 -> Add/2
  Add/1 -> Subtract/2, If Action Subsystem1/1(In1)
  Radians to Degrees/1 -> Add/1
  Constant/1 -> Subtract/1
  "Neck Head , Shoulder elbow2"/1 -> If Action Subsystem2/Action
  If Action Subsystem2/1(Out1) -> Out2/1
  Constant2/1 -> If Action Subsystem2/1(In1)
  In1/1 -> Trigonometric Function/1
  If Action Subsystem1/1(Out1) -> Out1/1
  "Neck Head , Shoulder elbow2"/2 -> If Action Subsystem1/Action
  In2/1 -> "Neck Head , Shoulder elbow2"/2
  Subtract/1 -> "Neck Head , Shoulder elbow2"/1

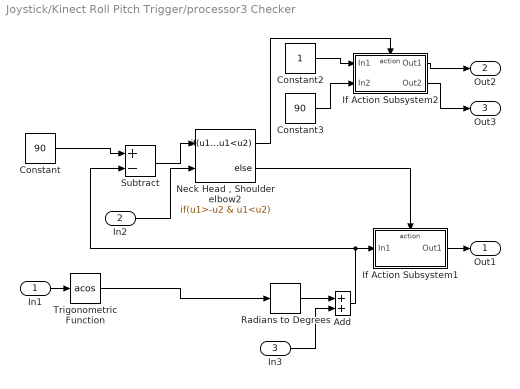
== system Joystick/Kinect Roll Pitch Trigger/processor3 Checker ==
  In1 : Inport
  In2 : Inport  Port=2
  In3 : Inport  Port=3
  Add : Sum
  Constant : Constant  Value=90
  Constant2 : Constant
  Constant3 : Constant  Value=90
  If Action Subsystem1 : Subsystem  TreatAsAtomicUnit=on
  If Action Subsystem2 : Subsystem  TreatAsAtomicUnit=on
  "Neck Head , Shoulder elbow2" : If  NumInputs=2  IfExpression=u1>-u2 & u1<u2
  Radians to Degrees : simulink_extras/Transformations/Radians to Degrees  SystemSampleTime=-1
  Subtract : Sum  Inputs=+-
  Trigonometric Function : Trigonometry  Operator=acos
  Out1 : Outport
  Out2 : Outport  Port=2
  Out3 : Outport  Port=3
  wires:
  If Action Subsystem2/2(Out2) -> Out3/1
  Constant3/1 -> If Action Subsystem2/2(In2)
  Trigonometric Function/1 -> Radians to Degrees/1
  In3/1 -> Add/2
  Add/1 -> Subtract/2, If Action Subsystem1/1(In1)
  Radians to Degrees/1 -> Add/1
  Constant/1 -> Subtract/1
  "Neck Head , Shoulder elbow2"/1 -> If Action Subsystem2/Action
  If Action Subsystem2/1(Out1) -> Out2/1
  Constant2/1 -> If Action Subsystem2/1(In1)
  In1/1 -> Trigonometric Function/1
  If Action Subsystem1/1(Out1) -> Out1/1
  "Neck Head , Shoulder elbow2"/2 -> If Action Subsystem1/Action
  In2/1 -> "Neck Head , Shoulder elbow2"/2
  Subtract/1 -> "Neck Head , Shoulder elbow2"/1

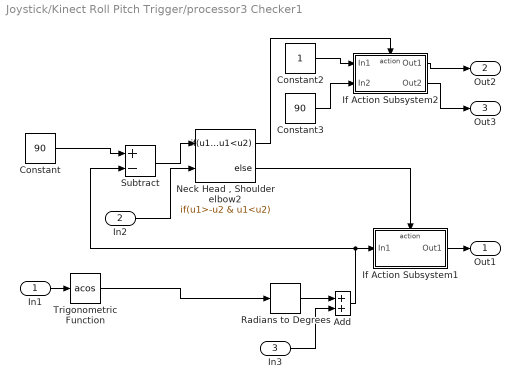
== system Joystick/Kinect Roll Pitch Trigger/processor3 Checker1 ==
  In1 : Inport
  In2 : Inport  Port=2
  In3 : Inport  Port=3
  Add : Sum
  Constant : Constant  Value=90
  Constant2 : Constant
  Constant3 : Constant  Value=90
  If Action Subsystem1 : Subsystem  TreatAsAtomicUnit=on
  If Action Subsystem2 : Subsystem  TreatAsAtomicUnit=on
  "Neck Head , Shoulder elbow2" : If  NumInputs=2  IfExpression=u1>-u2 & u1<u2
  Radians to Degrees : simulink_extras/Transformations/Radians to Degrees  SystemSampleTime=-1
  Subtract : Sum  Inputs=+-
  Trigonometric Function : Trigonometry  Operator=acos
  Out1 : Outport
  Out2 : Outport  Port=2
  Out3 : Outport  Port=3
  wires:
  If Action Subsystem2/2(Out2) -> Out3/1
  Constant3/1 -> If Action Subsystem2/2(In2)
  Trigonometric Function/1 -> Radians to Degrees/1
  In3/1 -> Add/2
  Add/1 -> Subtract/2, If Action Subsystem1/1(In1)
  Radians to Degrees/1 -> Add/1
  Constant/1 -> Subtract/1
  "Neck Head , Shoulder elbow2"/1 -> If Action Subsystem2/Action
  If Action Subsystem2/1(Out1) -> Out2/1
  Constant2/1 -> If Action Subsystem2/1(In1)
  In1/1 -> Trigonometric Function/1
  If Action Subsystem1/1(Out1) -> Out1/1
  "Neck Head , Shoulder elbow2"/2 -> If Action Subsystem1/Action
  In2/1 -> "Neck Head , Shoulder elbow2"/2
  Subtract/1 -> "Neck Head , Shoulder elbow2"/1

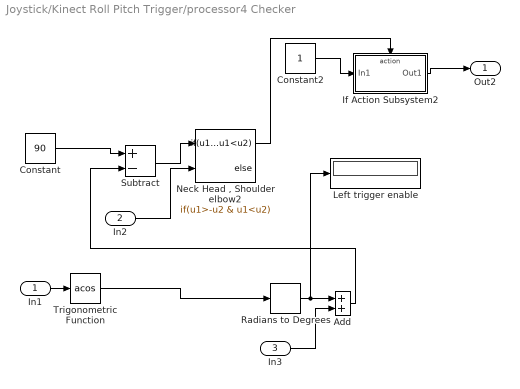
== system Joystick/Kinect Roll Pitch Trigger/processor4 Checker ==
  In1 : Inport
  In2 : Inport  Port=2
  In3 : Inport  Port=3
  Add : Sum
  Constant : Constant  Value=90
  Constant2 : Constant
  If Action Subsystem2 : Subsystem  TreatAsAtomicUnit=on
  Left trigger enable : Display
  "Neck Head , Shoulder elbow2" : If  NumInputs=2  IfExpression=u1>-u2 & u1<u2
  Radians to Degrees : simulink_extras/Transformations/Radians to Degrees  SystemSampleTime=-1
  Subtract : Sum  Inputs=+-
  Trigonometric Function : Trigonometry  Operator=acos
  Out2 : Outport
  wires:
  Subtract/1 -> "Neck Head , Shoulder elbow2"/1
  In2/1 -> "Neck Head , Shoulder elbow2"/2
  In1/1 -> Trigonometric Function/1
  Constant2/1 -> If Action Subsystem2/1(In1)
  If Action Subsystem2/1(Out1) -> Out2/1
  "Neck Head , Shoulder elbow2"/1 -> If Action Subsystem2/Action
  Constant/1 -> Subtract/1
  Radians to Degrees/1 -> Add/1, Left trigger enable/1
  Add/1 -> Subtract/2
  In3/1 -> Add/2
  Trigonometric Function/1 -> Radians to Degrees/1

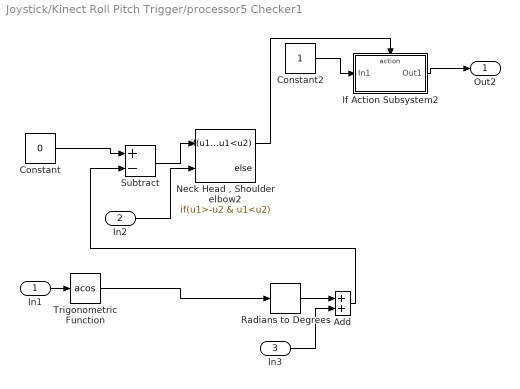
== system Joystick/Kinect Roll Pitch Trigger/processor5 Checker1 ==
  In1 : Inport
  In2 : Inport  Port=2
  In3 : Inport  Port=3
  Add : Sum
  Constant : Constant  Value=0
  Constant2 : Constant
  If Action Subsystem2 : Subsystem  TreatAsAtomicUnit=on
  "Neck Head , Shoulder elbow2" : If  NumInputs=2  IfExpression=u1>-u2 & u1<u2
  Radians to Degrees : simulink_extras/Transformations/Radians to Degrees  SystemSampleTime=-1
  Subtract : Sum  Inputs=+-
  Trigonometric Function : Trigonometry  Operator=acos
  Out2 : Outport
  wires:
  Subtract/1 -> "Neck Head , Shoulder elbow2"/1
  In2/1 -> "Neck Head , Shoulder elbow2"/2
  In1/1 -> Trigonometric Function/1
  Constant2/1 -> If Action Subsystem2/1(In1)
  If Action Subsystem2/1(Out1) -> Out2/1
  "Neck Head , Shoulder elbow2"/1 -> If Action Subsystem2/Action
  Constant/1 -> Subtract/1
  Radians to Degrees/1 -> Add/1
  Add/1 -> Subtract/2
  In3/1 -> Add/2
  Trigonometric Function/1 -> Radians to Degrees/1

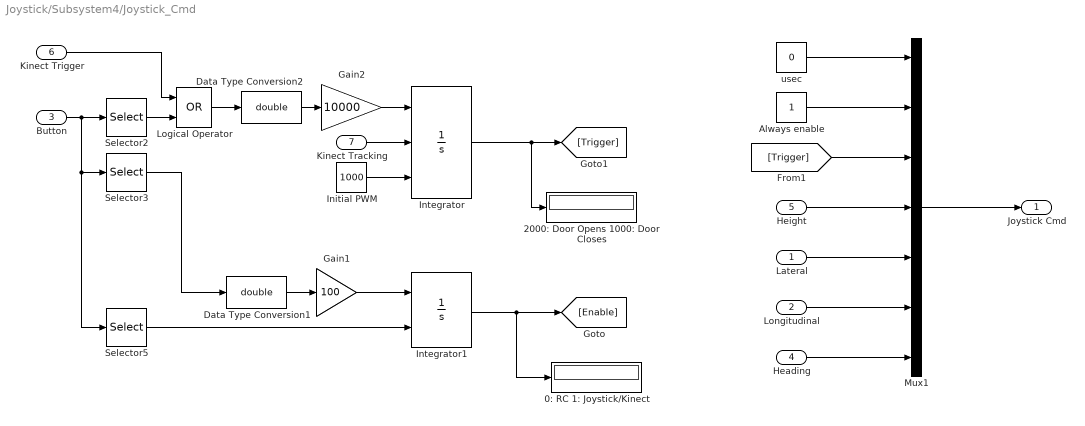
== system Joystick/Subsystem4/Joystick_Cmd ==
  Lateral : Inport
  Longitudinal : Inport  Port=2
  Button : Inport  Port=3
  Heading : Inport  Port=4
  Height : Inport  Port=5
  Kinect Trigger : Inport  Port=6
  Kinect Tracking : Inport  Port=7
  0: RC 1: Joystick/Kinect : Display
  2000: Door Opens 1000: Door Closes : Display
  Always enable : Constant  SampleTime=sample_time
  Data Type Conversion1 : DataTypeConversion  OutDataTypeStr=double
  Data Type Conversion2 : DataTypeConversion  OutDataTypeStr=double
  Gain1 : Gain  Gain=100
  Gain2 : Gain  Gain=10000
  Initial PWM : Constant  Value=1000
  Integrator : Integrator  ExternalReset=falling  InitialConditionSource=external  LimitOutput=on  UpperSaturationLimit=2000  LowerSaturationLimit=1000
  Integrator1 : Integrator  ExternalReset=either  LimitOutput=on  UpperSaturationLimit=1  LowerSaturationLimit=0
  Logical Operator : Logic  Operator=OR  AllPortsSameDT=off  OutDataTypeStr=boolean
  Mux1 : Mux  Inputs=7
  Selector2 : Selector  InputPortWidth=12  IndexOptions=Index vector (dialog)  Indices=1  OutputSizes=1
  Selector3 : Selector  InputPortWidth=12  IndexOptions=Index vector (dialog)  Indices=4  OutputSizes=1
  Selector5 : Selector  InputPortWidth=12  IndexOptions=Index vector (dialog)  Indices=3  OutputSizes=1
  usec : Constant  Value=0  SampleTime=sample_time
  Joystick Cmd : Outport
  wires:
  usec/1 -> Mux1/1
  Mux1/1 -> Joystick Cmd/1
  Height/1 -> Mux1/4
  Lateral/1 -> Mux1/5
  Longitudinal/1 -> Mux1/6
  Heading/1 -> Mux1/7
  Button/1 -> Selector2/1, Selector5/1, Selector3/1
  Initial PWM/1 -> Integrator/3
  Selector3/1 -> Data Type Conversion1/1
  Data Type Conversion1/1 -> Gain1/1
  Gain1/1 -> Integrator1/1
  Selector5/1 -> Integrator1/2
  [Trigger] -> Mux1/3
  Integrator/1 -> 2000: Door Opens 1000: Door Closes/1, [Trigger]
  Integrator1/1 -> [Enable], 0: RC 1: Joystick/Kinect/1
  Selector2/1 -> Logical Operator/2
  Kinect Trigger/1 -> Logical Operator/1
  Data Type Conversion2/1 -> Gain2/1
  Logical Operator/1 -> Data Type Conversion2/1
  Gain2/1 -> Integrator/1
  Always enable/1 -> Mux1/2
  Kinect Tracking/1 -> Integrator/2

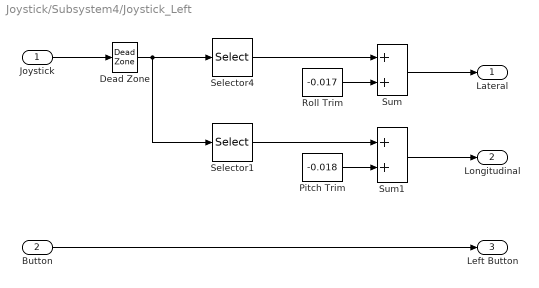
== system Joystick/Subsystem4/Joystick_Left ==
  Joystick : Inport
  Button : Inport  Port=2
  Dead Zone : DeadZone  LowerValue=-0.1  UpperValue=0.1  SaturateOnIntegerOverflow=on
  Pitch Trim : Constant  Value=-0.018
  Roll Trim : Constant  Value=-0.017
  Selector1 : Selector  InputPortWidth=4  IndexOptions=Index vector (dialog)  Indices=2  OutputSizes=1
  Selector4 : Selector  InputPortWidth=4  IndexOptions=Index vector (dialog)  Indices=1  OutputSizes=1
  Sum : Sum
  Sum1 : Sum
  Lateral : Outport
  Longitudinal : Outport  Port=2
  Left Button : Outport  Port=3
  wires:
  Joystick/1 -> Dead Zone/1
  Roll Trim/1 -> Sum/2
  Pitch Trim/1 -> Sum1/2
  Dead Zone/1 -> Selector4/1, Selector1/1
  Selector4/1 -> Sum/1
  Selector1/1 -> Sum1/1
  Sum/1 -> Lateral/1
  Sum1/1 -> Longitudinal/1
  Button/1 -> Left Button/1

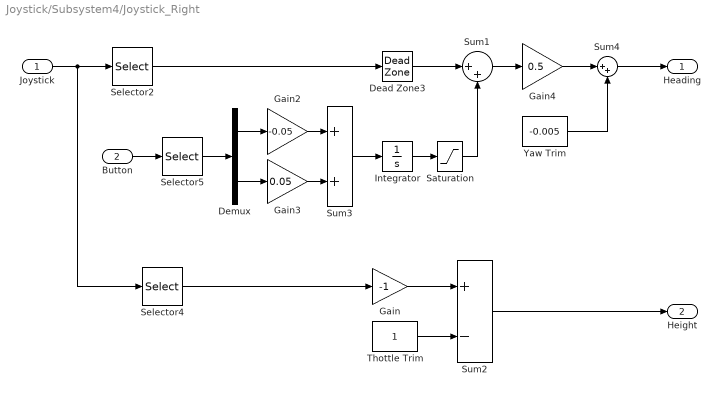
== system Joystick/Subsystem4/Joystick_Right ==
  Joystick : Inport
  Button : Inport  Port=2
  Dead Zone3 : DeadZone  LowerValue=-0.2  UpperValue=0.2  SaturateOnIntegerOverflow=on
  Demux : Demux  Outputs=2
  Gain : Gain  Gain=-1
  Gain2 : Gain  Gain=-0.05
  Gain3 : Gain  Gain=0.05
  Gain4 : Gain  Gain=0.5
  Integrator : Integrator
  Saturation : Saturate  UpperLimit=0.1  LowerLimit=-0.1
  Selector2 : Selector  InputPortWidth=3  IndexOptions=Index vector (dialog)  Indices=[1]  OutputSizes=1
  Selector4 : Selector  InputPortWidth=3  IndexOptions=Index vector (dialog)  Indices=2  OutputSizes=1
  Selector5 : Selector  InputPortWidth=11  IndexOptions=Index vector (dialog)  Indices=[4 5]  OutputSizes=1
  Sum1 : Sum  Inputs=|++
  Sum2 : Sum  Inputs=+-
  Sum3 : Sum  OutDataTypeStr=double
  Sum4 : Sum  Inputs=|++
  Thottle Trim : Constant
  Yaw Trim : Constant  Value=-0.005
  Heading : Outport
  Height : Outport  Port=2
  wires:
  Selector2/1 -> Dead Zone3/1
  Selector4/1 -> Gain/1
  Joystick/1 -> Selector2/1, Selector4/1
  Gain/1 -> Sum2/1
  Thottle Trim/1 -> Sum2/2
  Sum2/1 -> Height/1
  Button/1 -> Selector5/1
  Selector5/1 -> Demux/1
  Demux/2 -> Gain3/1
  Demux/1 -> Gain2/1
  Gain2/1 -> Sum3/1
  Gain3/1 -> Sum3/2
  Sum3/1 -> Integrator/1
  Dead Zone3/1 -> Sum1/1
  Integrator/1 -> Saturation/1
  Saturation/1 -> Sum1/2
  Gain4/1 -> Sum4/1
  Yaw Trim/1 -> Sum4/2
  Sum4/1 -> Heading/1
  Sum1/1 -> Gain4/1

== system Joystick/Subsystem4/Kinect Roll Pitch Trigger ==
  Kinect : Inport
  Kinect Tracking : Inport  Port=2
  Data Type Conversion : DataTypeConversion  OutDataTypeStr=boolean
  Demux : Demux  Outputs=3
  Scale sensitivity by one third1 : Gain  Gain=1/180
  Scale sensitivity by one third2 : Gain  Gain=1/180
  Scope1 : Scope
      settings: SaveName=ScopeData4
  Roll : Outport
  Pitch : Outport  Port=2
  Trigger : Outport  Port=3
  Tracking : Outport  Port=4
  wires:
  Kinect/1 -> Demux/1
  Demux/1 -> Scale sensitivity by one third1/1
  Demux/2 -> Scale sensitivity by one third2/1
  Demux/3 -> Trigger/1
  Scale sensitivity by one third1/1 -> Roll/1, Scope1/1
  Scale sensitivity by one third2/1 -> Pitch/1
  Kinect Tracking/1 -> Data Type Conversion/1
  Data Type Conversion/1 -> Tracking/1

== system Joystick/Kinect Roll Pitch Trigger/El-Sh, Ha-El Process2/Enabled Subsystem2 ==
  In1 : Inport
  Enable : EnablePort
  Out1 : Outport
  wires:
  In1/1 -> Out1/1

== system Joystick/Kinect Roll Pitch Trigger/He-Ne, El-Sh Process1/Enabled Subsystem1 ==
  In1 : Inport
  Enable : EnablePort
  Out1 : Outport
  wires:
  In1/1 -> Out1/1

== system Joystick/Kinect Roll Pitch Trigger/He-Ne, Ha-El Process3/Enabled Subsystem3 ==
  In1 : Inport
  Enable : EnablePort
  Out1 : Outport
  wires:
  In1/1 -> Out1/1

== system Joystick/Kinect Roll Pitch Trigger/He-Ne, LHa-Sh Process4/Enabled Subsystem1 ==
  In1 : Inport
  Enable : EnablePort
  Out1 : Outport
  wires:
  In1/1 -> Out1/1

== system Joystick/Kinect Roll Pitch Trigger/LEl-Sh, LHa-El Process5/Enabled Subsystem2 ==
  In1 : Inport
  Enable : EnablePort
  Out1 : Outport
  wires:
  In1/1 -> Out1/1

== system Joystick/Kinect Roll Pitch Trigger/processor1 Checker/If Action Subsystem1 ==
  In1 : Inport
  Action Port : ActionPort  ActionType=else
  Out1 : Outport  OutputWhenDisabled=reset  InitialOutput=[0.00000]
  wires:
  In1/1 -> Out1/1

== system Joystick/Kinect Roll Pitch Trigger/processor1 Checker/If Action Subsystem2 ==
  In1 : Inport
  In2 : Inport  Port=2
  Action Port : ActionPort  ActionType=then
  Out1 : Outport  OutputWhenDisabled=reset  InitialOutput=[0]
  Out2 : Outport  Port=2  OutputWhenDisabled=reset  InitialOutput=[0]
  wires:
  In2/1 -> Out2/1
  In1/1 -> Out1/1

== system Joystick/Kinect Roll Pitch Trigger/processor3 Checker/If Action Subsystem1 ==
  In1 : Inport
  Action Port : ActionPort  ActionType=else
  Out1 : Outport  OutputWhenDisabled=reset  InitialOutput=[0.00000]
  wires:
  In1/1 -> Out1/1

== system Joystick/Kinect Roll Pitch Trigger/processor3 Checker/If Action Subsystem2 ==
  In1 : Inport
  In2 : Inport  Port=2
  Action Port : ActionPort  ActionType=then
  Out1 : Outport  OutputWhenDisabled=reset  InitialOutput=[0]
  Out2 : Outport  Port=2  OutputWhenDisabled=reset  InitialOutput=[0]
  wires:
  In2/1 -> Out2/1
  In1/1 -> Out1/1

== system Joystick/Kinect Roll Pitch Trigger/processor3 Checker1/If Action Subsystem1 ==
  In1 : Inport
  Action Port : ActionPort  ActionType=else
  Out1 : Outport  OutputWhenDisabled=reset  InitialOutput=[0.00000]
  wires:
  In1/1 -> Out1/1

== system Joystick/Kinect Roll Pitch Trigger/processor3 Checker1/If Action Subsystem2 ==
  In1 : Inport
  In2 : Inport  Port=2
  Action Port : ActionPort  ActionType=then
  Out1 : Outport  OutputWhenDisabled=reset  InitialOutput=[0]
  Out2 : Outport  Port=2  OutputWhenDisabled=reset  InitialOutput=[0]
  wires:
  In2/1 -> Out2/1
  In1/1 -> Out1/1

== system Joystick/Kinect Roll Pitch Trigger/processor4 Checker/If Action Subsystem2 ==
  In1 : Inport
  Action Port : ActionPort  ActionType=then
  Out1 : Outport  OutputWhenDisabled=reset  InitialOutput=[0]
  wires:
  In1/1 -> Out1/1

== system Joystick/Kinect Roll Pitch Trigger/processor5 Checker1/If Action Subsystem2 ==
  In1 : Inport
  Action Port : ActionPort  ActionType=then
  Out1 : Outport  OutputWhenDisabled=reset  InitialOutput=[0]
  wires:
  In1/1 -> Out1/1

== matlab function Kinect Roll Pitch Trigger/Head Vector ==
  data: x input double; y input double; z input double; y1 output double
function y1 = fcn(x,y,z)
%#codegen
y1 = [x,y,z];

== matlab function Subsystem3/Process Flight Mode ==
  data: u input double; y output double
function y = fcn(u)
%#codegen

if u <=-0.5
    y = 0;  % Manual
elseif u>=0.5
    y = 2;  % Semi-autonomous
else
    y = 1;  % Stabilized
end

== matlab function Kinect Roll Pitch Trigger/Neck Vector ==
  data: x input double; y input double; z input double; y1 output double
function y1 = fcn(x,y,z)
%#codegen
y1 = [x,y,z];

== matlab function Kinect Roll Pitch Trigger/L shoulder Vector ==
  data: x input double; y input double; z input double; y1 output double
function y1 = fcn(x,y,z)
%#codegen
y1 = [x,y,z];

== matlab function Kinect Roll Pitch Trigger/L Hand Vector ==
  data: x input double; y input double; z input double; y1 output double
function y1 = fcn(x,y,z)
%#codegen
y1 = [x,y,z];

== matlab function Kinect Roll Pitch Trigger/L elbow Vector ==
  data: x input double; y input double; z input double; y1 output double
function y1 = fcn(x,y,z)
%#codegen
y1 = [x,y,z];

== matlab function Kinect Roll Pitch Trigger/R Hand Vector ==
  data: x input double; y input double; z input double; y1 output double
function y1 = fcn(x,y,z)
%#codegen
y1 = [x,y,z];

== matlab function Kinect Roll Pitch Trigger/R elbow ==
  data: x input double; y input double; z input double; y1 output double
function y1 = fcn(x,y,z)
%#codegen
y1 = [x,y,z];

== matlab function Kinect Roll Pitch Trigger/R shoulder ==
  data: x input double; y input double; z input double; y1 output double
function y1 = fcn(x,y,z)
%#codegen
y1 = [x,y,z];
